simulink model "test"  (R2022a)
settings: Solver=FixedStepDiscrete  StartTime=0.0  StopTime=inf  RelTol=1e-3  EnableMultiTasking=on
InitFcn:
  | run('busObjects.m')
undefined symbols (not defined in the file or in its folder): HS, IO291
libraries: aru_toolbox x14, speedgoatlib_IO691 x8, speedgoatlib_IO291 x1
settings Model: SimulationMode=external  ExtModeEnableFloating=off  Creator=Mechatronics  LastModifiedBy=Mechatronics
settings SolverCC: ConcurrentTasks=on  AlgebraicLoopSolver=TrustRegion  PositivePriorityOrder=on  InsertRTBMode=Never (minimum delay)
settings DataIOCC: SaveFormat=Array  SaveState=on  SignalLoggingName=logsOut
settings OptimizationCC: BlockReduction=off  BooleanDataType=off  OptimizeBlockIOStorage=off  BufferReuse=off  GlobalBufferReuse=off  ExpressionFolding=off  LocalBlockOutputs=off  InitFltsAndDblsToZero=on  OptimizeDataStoreBuffers=off  BusAssignmentInplaceUpdate=off
settings DebuggingCC: SaveWithParameterizedLinksMsg=none  UnderspecifiedInitializationDetection=Classic  MergeDetectMultiDrivingBlocksExec=none  CheckExecutionContextPreStartOutputMsg=on  SignalResolutionControl=TryResolveAllWithWarning  TasksWithSamePriorityMsg=none  UnconnectedInputMsg=warning  UnconnectedOutputMsg=warning  UnconnectedLineMsg=warning  SFUnexpectedBacktrackingDiag=warning  SFNoUnconditionalDefaultTransitionDiag=warning  SFExecutionAtInitializationDiag=none  SFMachineParentedDataDiag=warning  ArithmeticOperatorsInVariantConditions=warning
settings HardwareCC: ProdBitPerLong=64  ProdLongLongMode=on  ProdHWDeviceType=Intel->x86-64 (Linux 64)
settings ModelReferenceCC: PropagateSignalLabelsOutOfModel=off
settings SFSimCC: SimUseLocalCustomCode=off  SimTargetLang=C++
settings RTWCC: Description=Simulink Real-Time  SystemTargetFile=slrealtime.tlc  TemplateMakefile=slrealtime_default_tmf  RTWUseLocalCustomCode=off  Toolchain=Simulink Real-Time Toolchain  BuildConfiguration=Faster Runs  CodeExecutionProfiling=on  TargetLang=C++  DLArmComputeVersion=19.05
settings CodeAppCC: StateflowObjectComments=on
settings SimulinkRealTimeTargetCC: MATLABClassNameForMDSCustomization=Simulink.SoftwareTarget.GRTCustomization  UseGCCFastMath=on
settings ConfigComp: CovMetricSettings=dw  CovSaveCumulativeToWorkspaceVar=on  CovSaveSingleToWorkspaceVar=on  CovExternalEMLEnable=off  CovSFcnEnable=off

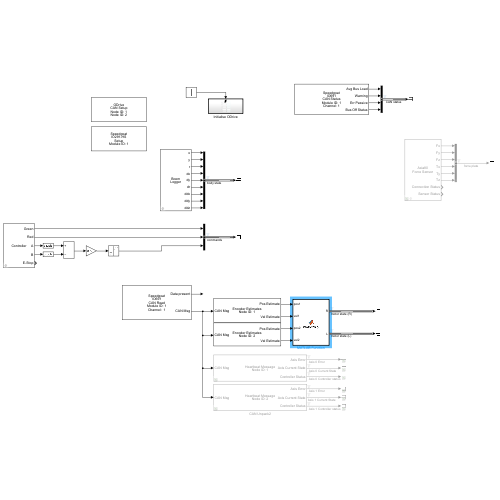
[thumbnail: Simulink's stored preview of the top-level diagram]
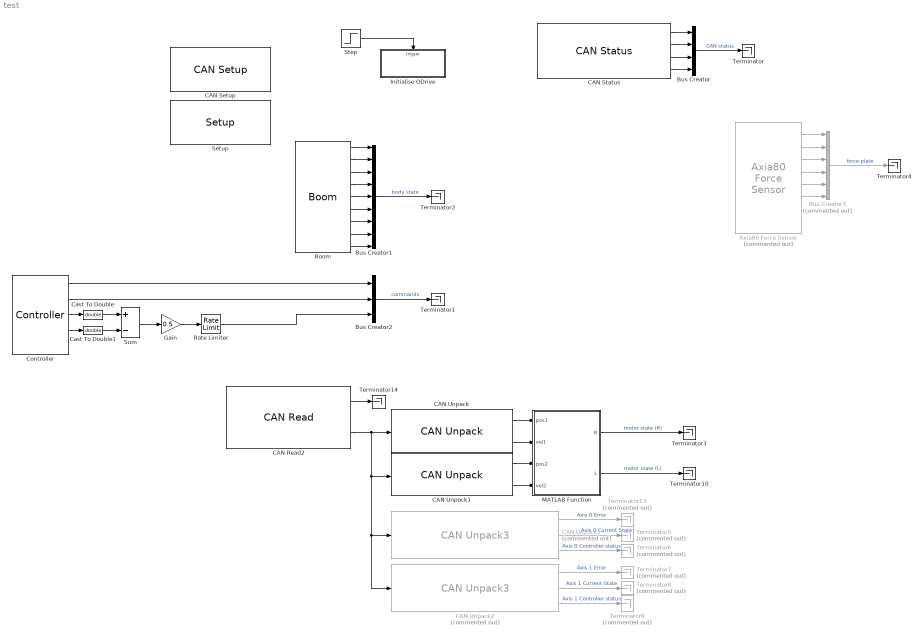
== system test ==
  Axia80 Force Sensor : aru_toolbox/Axia80 Force Sensor  Commented=on  resetBias=on  calibrationRangeParam=Range 0 (500N Fxy, 900N Fz, 20Nm Txyz)  sampleRateParam=975Hz  filterParam=No filtering (200Hz @ 0.5kHz, 350Hz @ 1kHz, 500Hz @ 2kHz, 1000Hz @ 4kHz)
      settings: SourceProductName=ARU Toolbox
  Boom : aru_toolbox/Boom  ts=0.001
      link override Serial Read HW FIFO: pciSlot=-1
      link override Serial Setup: pciSlot=-1
      settings: SourceProductName=ARU Toolbox
  Bus Creator : BusCreator  Inputs=4  OutDataTypeStr=Bus: CAN  NonVirtualBus=on
      settings: InheritFromInputs=off
  Bus Creator1 : BusCreator  Inputs=9  OutDataTypeStr=Bus: BodyState  NonVirtualBus=on
      settings: InheritFromInputs=off
  Bus Creator2 : BusCreator  Inputs=3  OutDataTypeStr=Bus: Command  NonVirtualBus=on
      settings: InheritFromInputs=off
  Bus Creator3 : BusCreator  Commented=on  Inputs=6  OutDataTypeStr=Bus: ForceData  NonVirtualBus=on
      settings: InheritFromInputs=off
  CAN Read2 : speedgoatlib_IO691/Legacy/CAN Read  id=1  ts=0.0005  channel=1  messageType=CAN  canType=CAN (HS)  BusOutput=off  initValues=[691 1 0.0005 0 1 1 0]
      settings: SourceProductName=Simulink Real-Time: Speedgoat Library
  CAN Setup : aru_toolbox/ODrive/CAN Setup  id1=1  id2=2
      settings: SourceProductName=Simulink Real-Time: Speedgoat I/O Blockset
  CAN Status : speedgoatlib_IO691/Legacy/CAN Status  moduleId=1  sampleTime=0.001  channel=1  busRecovery=Auto  arrayOutput=off  controllerCpuLoad=off  controllerLiveCount=off  initModeAct=off  avgBusLoad=on  receiving=off  RxQueueEmpty=off  dataOverrunRcv=off  rxBufferLevel=off  txPending=off  dataOverrunTx=off  txBufferLevel=off  errWarnLimit=on  errPassLimit=on  errBusOff=on  busRecoveryCounter=off  busCouplingErr=off  transceiverErr=off  opMode=off  brp=off  timeSegment1=off  timeSegment2=off  synchronisationJumpWidth=off  dataTSEG1=off  dataTSEG2=off  dataSJW=off  moduleType=691  qtyStatBlk=1  ptIdx=0  isFDMod=0
      settings: SourceProductName=Simulink Real-Time: Speedgoat I/O Blockset
  CAN Unpack : aru_toolbox/ODrive/CAN Unpack  id=1
      settings: SourceProductName=ARU Toolbox
  CAN Unpack1 : aru_toolbox/ODrive/CAN Unpack  id=2
      settings: SourceProductName=ARU Toolbox
  CAN Unpack2 : aru_toolbox/ODrive/CAN Unpack3  Commented=on  id=2
      settings: SourceProductName=ARU Toolbox
  CAN Unpack3 : aru_toolbox/ODrive/CAN Unpack3  Commented=on  id=1
      settings: SourceProductName=ARU Toolbox
  Cast To Double : DataTypeConversion  OutDataTypeStr=double  SaturateOnIntegerOverflow=off  RndMeth=Floor
  Cast To Double1 : DataTypeConversion  OutDataTypeStr=double  SaturateOnIntegerOverflow=off  RndMeth=Floor
  Controller : aru_toolbox/Controller
      settings: SourceProductName=ARU Toolbox
  Gain : Gain  Gain=0.5
  Initialise ODrive : Subsystem  TreatAsAtomicUnit=on
  MATLAB Function : MATLAB Function  TreatAsAtomicUnit=on
  Rate Limiter : RateLimiter  RisingSlewLimit=0.2  FallingSlewLimit=-0.2  SampleTimeMode=inherited
  "Setup " : speedgoatlib_IO291/Setup   parInternalModuleId=1  parPciSlot=-1  parModuleId=1  parModuleType=IO291-HS  parTtlDoChannels=[]  parTtlDoInitValues=1  parTtlDoReset=1  parTtlDiChannels=[1 2 3 4 5]  parIsolDiChannels=[]  parFetDoChannels=[1 2 3 4]  parFetDoInitValues=0  parFetDoReset=1
      settings: SourceProductName=Simulink Real-Time: Speedgoat I/O Blockset
  Step : Step  SampleTime=0
  Sum : Sum  Inputs=+-
  Terminator{,1..4,10,14} (7 alike) : Terminator
  Terminator{5..9,13} (6 alike) : Terminator  Commented=on
  wires:
  Step/1 -> Initialise ODrive/Trigger
  CAN Unpack/1 -> MATLAB Function/1(pos1)
  CAN Unpack/2 -> MATLAB Function/2(vel1)
  CAN Unpack1/1 -> MATLAB Function/3(pos2)
  CAN Unpack1/2 -> MATLAB Function/4(vel2)
  CAN Read2/2 -> CAN Unpack2/1, CAN Unpack3/1, CAN Unpack1/1, CAN Unpack/1
  CAN Status/1 -> Bus Creator/1
  CAN Status/2 -> Bus Creator/2
  CAN Status/3 -> Bus Creator/3
  CAN Status/4 -> Bus Creator/4
  CAN Unpack3/1 -> Terminator13/1  "Axis 0 Error"
  CAN Unpack3/2 -> Terminator5/1  "Axis 0 Current State"
  CAN Unpack3/3 -> Terminator6/1  "Axis 0 Controller status"
  CAN Unpack2/1 -> Terminator7/1  "Axis 1 Error"
  CAN Unpack2/2 -> Terminator8/1  "Axis 1 Current State"
  CAN Unpack2/3 -> Terminator9/1  "Axis 1 Controller status"
  CAN Read2/1 -> Terminator14/1
  MATLAB Function/1(R) -> Terminator3/1  "motor state (R)"
  MATLAB Function/2(L) -> Terminator10/1  "motor state (L)"
  Bus Creator/1 -> Terminator/1  "CAN status"
  Boom/1 -> Bus Creator1/1
  Boom/9 -> Bus Creator1/9
  Boom/2 -> Bus Creator1/2
  Boom/3 -> Bus Creator1/3
  Boom/4 -> Bus Creator1/4
  Boom/5 -> Bus Creator1/5
  Boom/6 -> Bus Creator1/6
  Boom/7 -> Bus Creator1/7
  Boom/8 -> Bus Creator1/8
  Bus Creator1/1 -> Terminator2/1  "body state"
  Controller/1 -> Bus Creator2/1
  Controller/2 -> Bus Creator2/2
  Axia80 Force Sensor/1 -> Bus Creator3/1
  Axia80 Force Sensor/6 -> Bus Creator3/6
  Axia80 Force Sensor/5 -> Bus Creator3/5
  Axia80 Force Sensor/4 -> Bus Creator3/4
  Axia80 Force Sensor/3 -> Bus Creator3/3
  Axia80 Force Sensor/2 -> Bus Creator3/2
  Bus Creator3/1 -> Terminator4/1  "force plate"
  Controller/3 -> Cast To Double/1
  Controller/4 -> Cast To Double1/1
  Cast To Double/1 -> Sum/1
  Cast To Double1/1 -> Sum/2
  Sum/1 -> Gain/1
  Gain/1 -> Rate Limiter/1
  Rate Limiter/1 -> Bus Creator2/3
  Bus Creator2/1 -> Terminator1/1  "commands"

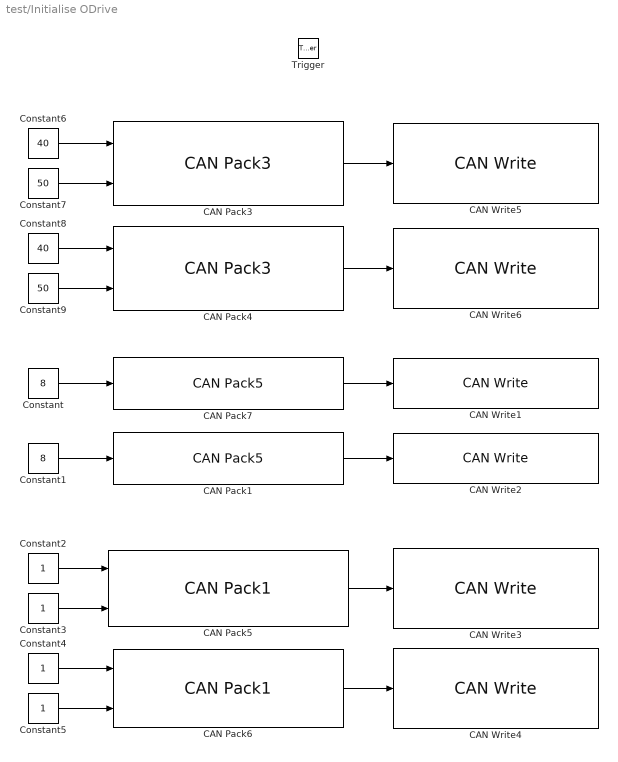
== system test/Initialise ODrive ==
  Trigger : TriggerPort  VariantControl=Variant
  CAN Pack1 : aru_toolbox/ODrive/CAN Pack5  id=2
      settings: SourceProductName=ARU Toolbox
  CAN Pack3 : aru_toolbox/ODrive/CAN Pack3  id=1
      settings: SourceProductName=ARU Toolbox
  CAN Pack4 : aru_toolbox/ODrive/CAN Pack3  id=2
      settings: SourceProductName=ARU Toolbox
  CAN Pack5 : aru_toolbox/ODrive/CAN Pack1  id=1
      settings: SourceProductName=ARU Toolbox
  CAN Pack6 : aru_toolbox/ODrive/CAN Pack1  id=2
      settings: SourceProductName=ARU Toolbox
  CAN Pack7 : aru_toolbox/ODrive/CAN Pack5  id=1
      settings: SourceProductName=ARU Toolbox
  CAN Write{1..6} (6 alike) : speedgoatlib_IO691/Legacy/CAN Write  id=1  ts=-1  channel=1  messageType=CAN  BusInput=off  enableStatusPort=off  canType=CAN (HS)  initValues=[691 1 -1 0 1 1 0 0]
      settings: SourceProductName=Simulink Real-Time: Speedgoat I/O Blockset
  Constant : Constant  Value=8
  Constant1 : Constant  Value=8
  Constant2 : Constant  OutDataTypeStr=int32
  Constant3 : Constant
  Constant4 : Constant
  Constant5 : Constant
  Constant6 : Constant  Value=40
  Constant7 : Constant  Value=50
  Constant8 : Constant  Value=40
  Constant9 : Constant  Value=50
  wires:
  CAN Pack7/1 -> CAN Write1/1
  Constant/1 -> CAN Pack7/1
  CAN Pack1/1 -> CAN Write2/1
  Constant1/1 -> CAN Pack1/1
  Constant3/1 -> CAN Pack5/2
  Constant2/1 -> CAN Pack5/1
  Constant4/1 -> CAN Pack6/1
  Constant5/1 -> CAN Pack6/2
  CAN Pack5/1 -> CAN Write3/1
  CAN Pack6/1 -> CAN Write4/1
  Constant7/1 -> CAN Pack3/2
  Constant6/1 -> CAN Pack3/1
  Constant8/1 -> CAN Pack4/1
  Constant9/1 -> CAN Pack4/2
  CAN Pack3/1 -> CAN Write5/1
  CAN Pack4/1 -> CAN Write6/1

== matlab function test/MATLAB Function ==
  data: pos1 input; R output Bus: MotorState; vel1 input; pos2 input; vel2 input; L output Bus: MotorState
function [R,L] = motor2hip(pos1, vel1, pos2, vel2) %#codegen
N = 6;
femurTaper = 0.080111; %rad

actualR = -0.2971;
actualL = -0.0555;

offsetR = femurTaper - actualR;
offsetL = pi - femurTaper - actualL;

% offsetR = 0;
% offsetL = 0;
% ODrive uses units turns and turns/s so need to explicity convert to
% radians
R.q = pos1*2*pi/N + offsetR;
R.w = vel1*2*pi/N;
L.q = pos2*2*pi/N + offsetL;
L.w = vel2*2*pi/N;
end
